simulink model "multi_opts"  (Simulink 4.00)
settings: Solver=ode45  SolverMode=SingleTasking  StartTime=0  StopTime=5  MaxStep=0.1  RelTol=1e-3  AbsTol=1e-3
libraries: simulink3 x3
(part 2 of 2)

== system multi_opts/GPe/2 input channel3/leaky integration ==
  Inport : Inport  Port=1  LatchInput=off
  Gain : Gain  Gain=A_rate  Multiplication=Element-wise(K.*u)  SaturateOnIntegerOverflow=on
  Integrator : Integrator  ExternalReset=none  InitialConditionSource=internal  InitialCondition=0  LimitOutput=off  UpperSaturationLimit=inf  LowerSaturationLimit=-inf  ShowSaturationPort=off  ShowStatePort=off  AbsoluteTolerance=auto
  decay const : Gain  Orientation=left  Gain=-A_rate  Multiplication=Element-wise(K.*u)  SaturateOnIntegerOverflow=on
  sum : Sum  Inputs=++  SaturateOnIntegerOverflow=on
  Outport : Outport  Port=1  InitialOutput=0
  wires:
  decay const/1 -> sum/2
  sum/1 -> Integrator/1
  Integrator/1 -> Outport/1, decay const/1
  Inport/1 -> Gain/1
  Gain/1 -> sum/1

== system multi_opts/GPe/2 input channel4/input summation ==
  x1 : Inport  Port=1  LatchInput=off
  x2 : Inport  Port=2  LatchInput=off
  Sum : Sum  Inputs=++  SaturateOnIntegerOverflow=on
  W1 : Gain  Gain=W_str  Multiplication=Element-wise(K.*u)  SaturateOnIntegerOverflow=on
  W2 : Gain  Gain=W_STN  Multiplication=Element-wise(K.*u)  SaturateOnIntegerOverflow=on
  out_1 : Outport  Port=1  InitialOutput=0
  wires:
  W2/1 -> Sum/2
  W1/1 -> Sum/1
  x2/1 -> W2/1
  x1/1 -> W1/1
  Sum/1 -> out_1/1

== system multi_opts/GPe/2 input channel4/leaky integration ==
  Inport : Inport  Port=1  LatchInput=off
  Gain : Gain  Gain=A_rate  Multiplication=Element-wise(K.*u)  SaturateOnIntegerOverflow=on
  Integrator : Integrator  ExternalReset=none  InitialConditionSource=internal  InitialCondition=0  LimitOutput=off  UpperSaturationLimit=inf  LowerSaturationLimit=-inf  ShowSaturationPort=off  ShowStatePort=off  AbsoluteTolerance=auto
  decay const : Gain  Orientation=left  Gain=-A_rate  Multiplication=Element-wise(K.*u)  SaturateOnIntegerOverflow=on
  sum : Sum  Inputs=++  SaturateOnIntegerOverflow=on
  Outport : Outport  Port=1  InitialOutput=0
  wires:
  Gain/1 -> sum/1
  Inport/1 -> Gain/1
  Integrator/1 -> decay const/1, Outport/1
  sum/1 -> Integrator/1
  decay const/1 -> sum/2

== system multi_opts/GPe/2 input channel5/input summation ==
  x1 : Inport  Port=1  LatchInput=off
  x2 : Inport  Port=2  LatchInput=off
  Sum : Sum  Inputs=++  SaturateOnIntegerOverflow=on
  W1 : Gain  Gain=W_str  Multiplication=Element-wise(K.*u)  SaturateOnIntegerOverflow=on
  W2 : Gain  Gain=W_STN  Multiplication=Element-wise(K.*u)  SaturateOnIntegerOverflow=on
  out_1 : Outport  Port=1  InitialOutput=0
  wires:
  Sum/1 -> out_1/1
  x1/1 -> W1/1
  x2/1 -> W2/1
  W1/1 -> Sum/1
  W2/1 -> Sum/2

== system multi_opts/GPe/2 input channel5/leaky integration ==
  Inport : Inport  Port=1  LatchInput=off
  Gain : Gain  Gain=A_rate  Multiplication=Element-wise(K.*u)  SaturateOnIntegerOverflow=on
  Integrator : Integrator  ExternalReset=none  InitialConditionSource=internal  InitialCondition=0  LimitOutput=off  UpperSaturationLimit=inf  LowerSaturationLimit=-inf  ShowSaturationPort=off  ShowStatePort=off  AbsoluteTolerance=auto
  decay const : Gain  Orientation=left  Gain=-A_rate  Multiplication=Element-wise(K.*u)  SaturateOnIntegerOverflow=on
  sum : Sum  Inputs=++  SaturateOnIntegerOverflow=on
  Outport : Outport  Port=1  InitialOutput=0
  wires:
  decay const/1 -> sum/2
  sum/1 -> Integrator/1
  Integrator/1 -> Outport/1, decay const/1
  Inport/1 -> Gain/1
  Gain/1 -> sum/1

== system multi_opts/GPi/2 input channel/input summation ==
  x1 : Inport  Port=1  LatchInput=off
  x2 : Inport  Port=2  LatchInput=off
  x3 : Inport  Port=3  LatchInput=off
  Sum : Sum  Inputs=+++  SaturateOnIntegerOverflow=on
  W1 : Gain  Gain=W_str  Multiplication=Element-wise(K.*u)  SaturateOnIntegerOverflow=on
  W2 : Gain  Gain=W_STN  Multiplication=Element-wise(K.*u)  SaturateOnIntegerOverflow=on
  W3 : Gain  Gain=W_GPe  Multiplication=Element-wise(K.*u)  SaturateOnIntegerOverflow=on
  out_1 : Outport  Port=1  InitialOutput=0
  wires:
  Sum/1 -> out_1/1
  x1/1 -> W1/1
  x2/1 -> W2/1
  W1/1 -> Sum/1
  W2/1 -> Sum/2
  x3/1 -> W3/1
  W3/1 -> Sum/3

== system multi_opts/GPi/2 input channel/leaky integration ==
  Inport : Inport  Port=1  LatchInput=off
  Gain : Gain  Gain=A_rate  Multiplication=Element-wise(K.*u)  SaturateOnIntegerOverflow=on
  Integrator : Integrator  ExternalReset=none  InitialConditionSource=internal  InitialCondition=0  LimitOutput=off  UpperSaturationLimit=inf  LowerSaturationLimit=-inf  ShowSaturationPort=off  ShowStatePort=off  AbsoluteTolerance=auto
  decay const : Gain  Orientation=left  Gain=-A_rate  Multiplication=Element-wise(K.*u)  SaturateOnIntegerOverflow=on
  sum : Sum  Inputs=++  SaturateOnIntegerOverflow=on
  Outport : Outport  Port=1  InitialOutput=0
  wires:
  decay const/1 -> sum/2
  sum/1 -> Integrator/1
  Integrator/1 -> Outport/1, decay const/1
  Inport/1 -> Gain/1
  Gain/1 -> sum/1

== system multi_opts/GPi/2 input channel1/input summation ==
  x1 : Inport  Port=1  LatchInput=off
  x2 : Inport  Port=2  LatchInput=off
  x3 : Inport  Port=3  LatchInput=off
  Sum : Sum  Inputs=+++  SaturateOnIntegerOverflow=on
  W1 : Gain  Gain=W_str  Multiplication=Element-wise(K.*u)  SaturateOnIntegerOverflow=on
  W2 : Gain  Gain=W_STN  Multiplication=Element-wise(K.*u)  SaturateOnIntegerOverflow=on
  W3 : Gain  Gain=W_GPe  Multiplication=Element-wise(K.*u)  SaturateOnIntegerOverflow=on
  out_1 : Outport  Port=1  InitialOutput=0
  wires:
  W3/1 -> Sum/3
  x3/1 -> W3/1
  W2/1 -> Sum/2
  W1/1 -> Sum/1
  x2/1 -> W2/1
  x1/1 -> W1/1
  Sum/1 -> out_1/1

== system multi_opts/GPi/2 input channel1/leaky integration ==
  Inport : Inport  Port=1  LatchInput=off
  Gain : Gain  Gain=A_rate  Multiplication=Element-wise(K.*u)  SaturateOnIntegerOverflow=on
  Integrator : Integrator  ExternalReset=none  InitialConditionSource=internal  InitialCondition=0  LimitOutput=off  UpperSaturationLimit=inf  LowerSaturationLimit=-inf  ShowSaturationPort=off  ShowStatePort=off  AbsoluteTolerance=auto
  decay const : Gain  Orientation=left  Gain=-A_rate  Multiplication=Element-wise(K.*u)  SaturateOnIntegerOverflow=on
  sum : Sum  Inputs=++  SaturateOnIntegerOverflow=on
  Outport : Outport  Port=1  InitialOutput=0
  wires:
  Gain/1 -> sum/1
  Inport/1 -> Gain/1
  Integrator/1 -> decay const/1, Outport/1
  sum/1 -> Integrator/1
  decay const/1 -> sum/2

== system multi_opts/GPi/2 input channel2/input summation ==
  x1 : Inport  Port=1  LatchInput=off
  x2 : Inport  Port=2  LatchInput=off
  x3 : Inport  Port=3  LatchInput=off
  Sum : Sum  Inputs=+++  SaturateOnIntegerOverflow=on
  W1 : Gain  Gain=W_str  Multiplication=Element-wise(K.*u)  SaturateOnIntegerOverflow=on
  W2 : Gain  Gain=W_STN  Multiplication=Element-wise(K.*u)  SaturateOnIntegerOverflow=on
  W3 : Gain  Gain=W_GPe  Multiplication=Element-wise(K.*u)  SaturateOnIntegerOverflow=on
  out_1 : Outport  Port=1  InitialOutput=0
  wires:
  Sum/1 -> out_1/1
  x1/1 -> W1/1
  x2/1 -> W2/1
  W1/1 -> Sum/1
  W2/1 -> Sum/2
  x3/1 -> W3/1
  W3/1 -> Sum/3

== system multi_opts/GPi/2 input channel2/leaky integration ==
  Inport : Inport  Port=1  LatchInput=off
  Gain : Gain  Gain=A_rate  Multiplication=Element-wise(K.*u)  SaturateOnIntegerOverflow=on
  Integrator : Integrator  ExternalReset=none  InitialConditionSource=internal  InitialCondition=0  LimitOutput=off  UpperSaturationLimit=inf  LowerSaturationLimit=-inf  ShowSaturationPort=off  ShowStatePort=off  AbsoluteTolerance=auto
  decay const : Gain  Orientation=left  Gain=-A_rate  Multiplication=Element-wise(K.*u)  SaturateOnIntegerOverflow=on
  sum : Sum  Inputs=++  SaturateOnIntegerOverflow=on
  Outport : Outport  Port=1  InitialOutput=0
  wires:
  decay const/1 -> sum/2
  sum/1 -> Integrator/1
  Integrator/1 -> Outport/1, decay const/1
  Inport/1 -> Gain/1
  Gain/1 -> sum/1

== system multi_opts/GPi/2 input channel3/input summation ==
  x1 : Inport  Port=1  LatchInput=off
  x2 : Inport  Port=2  LatchInput=off
  x3 : Inport  Port=3  LatchInput=off
  Sum : Sum  Inputs=+++  SaturateOnIntegerOverflow=on
  W1 : Gain  Gain=W_str  Multiplication=Element-wise(K.*u)  SaturateOnIntegerOverflow=on
  W2 : Gain  Gain=W_STN  Multiplication=Element-wise(K.*u)  SaturateOnIntegerOverflow=on
  W3 : Gain  Gain=W_GPe  Multiplication=Element-wise(K.*u)  SaturateOnIntegerOverflow=on
  out_1 : Outport  Port=1  InitialOutput=0
  wires:
  W3/1 -> Sum/3
  x3/1 -> W3/1
  W2/1 -> Sum/2
  W1/1 -> Sum/1
  x2/1 -> W2/1
  x1/1 -> W1/1
  Sum/1 -> out_1/1

== system multi_opts/GPi/2 input channel3/leaky integration ==
  Inport : Inport  Port=1  LatchInput=off
  Gain : Gain  Gain=A_rate  Multiplication=Element-wise(K.*u)  SaturateOnIntegerOverflow=on
  Integrator : Integrator  ExternalReset=none  InitialConditionSource=internal  InitialCondition=0  LimitOutput=off  UpperSaturationLimit=inf  LowerSaturationLimit=-inf  ShowSaturationPort=off  ShowStatePort=off  AbsoluteTolerance=auto
  decay const : Gain  Orientation=left  Gain=-A_rate  Multiplication=Element-wise(K.*u)  SaturateOnIntegerOverflow=on
  sum : Sum  Inputs=++  SaturateOnIntegerOverflow=on
  Outport : Outport  Port=1  InitialOutput=0
  wires:
  Gain/1 -> sum/1
  Inport/1 -> Gain/1
  Integrator/1 -> decay const/1, Outport/1
  sum/1 -> Integrator/1
  decay const/1 -> sum/2

== system multi_opts/GPi/2 input channel4/input summation ==
  x1 : Inport  Port=1  LatchInput=off
  x2 : Inport  Port=2  LatchInput=off
  x3 : Inport  Port=3  LatchInput=off
  Sum : Sum  Inputs=+++  SaturateOnIntegerOverflow=on
  W1 : Gain  Gain=W_str  Multiplication=Element-wise(K.*u)  SaturateOnIntegerOverflow=on
  W2 : Gain  Gain=W_STN  Multiplication=Element-wise(K.*u)  SaturateOnIntegerOverflow=on
  W3 : Gain  Gain=W_GPe  Multiplication=Element-wise(K.*u)  SaturateOnIntegerOverflow=on
  out_1 : Outport  Port=1  InitialOutput=0
  wires:
  Sum/1 -> out_1/1
  x1/1 -> W1/1
  x2/1 -> W2/1
  W1/1 -> Sum/1
  W2/1 -> Sum/2
  x3/1 -> W3/1
  W3/1 -> Sum/3

== system multi_opts/GPi/2 input channel4/leaky integration ==
  Inport : Inport  Port=1  LatchInput=off
  Gain : Gain  Gain=A_rate  Multiplication=Element-wise(K.*u)  SaturateOnIntegerOverflow=on
  Integrator : Integrator  ExternalReset=none  InitialConditionSource=internal  InitialCondition=0  LimitOutput=off  UpperSaturationLimit=inf  LowerSaturationLimit=-inf  ShowSaturationPort=off  ShowStatePort=off  AbsoluteTolerance=auto
  decay const : Gain  Orientation=left  Gain=-A_rate  Multiplication=Element-wise(K.*u)  SaturateOnIntegerOverflow=on
  sum : Sum  Inputs=++  SaturateOnIntegerOverflow=on
  Outport : Outport  Port=1  InitialOutput=0
  wires:
  decay const/1 -> sum/2
  sum/1 -> Integrator/1
  Integrator/1 -> Outport/1, decay const/1
  Inport/1 -> Gain/1
  Gain/1 -> sum/1

== system multi_opts/GPi/2 input channel5/input summation ==
  x1 : Inport  Port=1  LatchInput=off
  x2 : Inport  Port=2  LatchInput=off
  x3 : Inport  Port=3  LatchInput=off
  Sum : Sum  Inputs=+++  SaturateOnIntegerOverflow=on
  W1 : Gain  Gain=W_str  Multiplication=Element-wise(K.*u)  SaturateOnIntegerOverflow=on
  W2 : Gain  Gain=W_STN  Multiplication=Element-wise(K.*u)  SaturateOnIntegerOverflow=on
  W3 : Gain  Gain=W_GPe  Multiplication=Element-wise(K.*u)  SaturateOnIntegerOverflow=on
  out_1 : Outport  Port=1  InitialOutput=0
  wires:
  W3/1 -> Sum/3
  x3/1 -> W3/1
  W2/1 -> Sum/2
  W1/1 -> Sum/1
  x2/1 -> W2/1
  x1/1 -> W1/1
  Sum/1 -> out_1/1

== system multi_opts/GPi/2 input channel5/leaky integration ==
  Inport : Inport  Port=1  LatchInput=off
  Gain : Gain  Gain=A_rate  Multiplication=Element-wise(K.*u)  SaturateOnIntegerOverflow=on
  Integrator : Integrator  ExternalReset=none  InitialConditionSource=internal  InitialCondition=0  LimitOutput=off  UpperSaturationLimit=inf  LowerSaturationLimit=-inf  ShowSaturationPort=off  ShowStatePort=off  AbsoluteTolerance=auto
  decay const : Gain  Orientation=left  Gain=-A_rate  Multiplication=Element-wise(K.*u)  SaturateOnIntegerOverflow=on
  sum : Sum  Inputs=++  SaturateOnIntegerOverflow=on
  Outport : Outport  Port=1  InitialOutput=0
  wires:
  Gain/1 -> sum/1
  Inport/1 -> Gain/1
  Integrator/1 -> decay const/1, Outport/1
  sum/1 -> Integrator/1
  decay const/1 -> sum/2

== system multi_opts/STN/STN discrete model/2 input channel ==
  Cortex : Inport  Orientation=down  Port=1  LatchInput=off
  GPe : Inport  Orientation=down  Port=2  LatchInput=off
  input summation : Subsystem  Orientation=down
      settings: RTWFcnNameOpts=Auto  RTWFileNameOpts=Auto
  leaky integration : Subsystem  Orientation=down
      settings: RTWFcnNameOpts=Auto  RTWFileNameOpts=Auto
  piecewise lin. : S-Function  Orientation=down  FunctionName=Mpieclin  Parameters=slope,thresh  PortCounts=[]  SFunctionModules=''
  out : Outport  Orientation=down  Port=1  InitialOutput=0
  wires:
  piecewise lin./1 -> out/1
  GPe/1 -> input summation/2(x2)
  Cortex/1 -> input summation/1(x1)
  leaky integration/1(Outport) -> piecewise lin./1
  input summation/1(out_1) -> leaky integration/1(Inport)

== system multi_opts/STN/STN discrete model/2 input channel1 ==
  Cortex : Inport  Orientation=down  Port=1  LatchInput=off
  GPe : Inport  Orientation=down  Port=2  LatchInput=off
  input summation : Subsystem  Orientation=down
      settings: RTWFcnNameOpts=Auto  RTWFileNameOpts=Auto
  leaky integration : Subsystem  Orientation=down
      settings: RTWFcnNameOpts=Auto  RTWFileNameOpts=Auto
  piecewise lin. : S-Function  Orientation=down  FunctionName=Mpieclin  Parameters=slope,thresh  PortCounts=[]  SFunctionModules=''
  out : Outport  Orientation=down  Port=1  InitialOutput=0
  wires:
  input summation/1(out_1) -> leaky integration/1(Inport)
  leaky integration/1(Outport) -> piecewise lin./1
  Cortex/1 -> input summation/1(x1)
  GPe/1 -> input summation/2(x2)
  piecewise lin./1 -> out/1

== system multi_opts/STN/STN discrete model/2 input channel2 ==
  Cortex : Inport  Orientation=down  Port=1  LatchInput=off
  GPe : Inport  Orientation=down  Port=2  LatchInput=off
  input summation : Subsystem  Orientation=down
      settings: RTWFcnNameOpts=Auto  RTWFileNameOpts=Auto
  leaky integration : Subsystem  Orientation=down
      settings: RTWFcnNameOpts=Auto  RTWFileNameOpts=Auto
  piecewise lin. : S-Function  Orientation=down  FunctionName=Mpieclin  Parameters=slope,thresh  PortCounts=[]  SFunctionModules=''
  out : Outport  Orientation=down  Port=1  InitialOutput=0
  wires:
  piecewise lin./1 -> out/1
  GPe/1 -> input summation/2(x2)
  Cortex/1 -> input summation/1(x1)
  leaky integration/1(Outport) -> piecewise lin./1
  input summation/1(out_1) -> leaky integration/1(Inport)

== system multi_opts/STN/STN discrete model/2 input channel3 ==
  Cortex : Inport  Orientation=down  Port=1  LatchInput=off
  GPe : Inport  Orientation=down  Port=2  LatchInput=off
  input summation : Subsystem  Orientation=down
      settings: RTWFcnNameOpts=Auto  RTWFileNameOpts=Auto
  leaky integration : Subsystem  Orientation=down
      settings: RTWFcnNameOpts=Auto  RTWFileNameOpts=Auto
  piecewise lin. : S-Function  Orientation=down  FunctionName=Mpieclin  Parameters=slope,thresh  PortCounts=[]  SFunctionModules=''
  out : Outport  Orientation=down  Port=1  InitialOutput=0
  wires:
  input summation/1(out_1) -> leaky integration/1(Inport)
  leaky integration/1(Outport) -> piecewise lin./1
  Cortex/1 -> input summation/1(x1)
  GPe/1 -> input summation/2(x2)
  piecewise lin./1 -> out/1

== system multi_opts/STN/STN discrete model/2 input channel4 ==
  Cortex : Inport  Orientation=down  Port=1  LatchInput=off
  GPe : Inport  Orientation=down  Port=2  LatchInput=off
  input summation : Subsystem  Orientation=down
      settings: RTWFcnNameOpts=Auto  RTWFileNameOpts=Auto
  leaky integration : Subsystem  Orientation=down
      settings: RTWFcnNameOpts=Auto  RTWFileNameOpts=Auto
  piecewise lin. : S-Function  Orientation=down  FunctionName=Mpieclin  Parameters=slope,thresh  PortCounts=[]  SFunctionModules=''
  out : Outport  Orientation=down  Port=1  InitialOutput=0
  wires:
  piecewise lin./1 -> out/1
  GPe/1 -> input summation/2(x2)
  Cortex/1 -> input summation/1(x1)
  leaky integration/1(Outport) -> piecewise lin./1
  input summation/1(out_1) -> leaky integration/1(Inport)

== system multi_opts/STN/STN discrete model/2 input channel5 ==
  Cortex : Inport  Orientation=down  Port=1  LatchInput=off
  GPe : Inport  Orientation=down  Port=2  LatchInput=off
  input summation : Subsystem  Orientation=down
      settings: RTWFcnNameOpts=Auto  RTWFileNameOpts=Auto
  leaky integration : Subsystem  Orientation=down
      settings: RTWFcnNameOpts=Auto  RTWFileNameOpts=Auto
  piecewise lin. : S-Function  Orientation=down  FunctionName=Mpieclin  Parameters=slope,thresh  PortCounts=[]  SFunctionModules=''
  out : Outport  Orientation=down  Port=1  InitialOutput=0
  wires:
  input summation/1(out_1) -> leaky integration/1(Inport)
  leaky integration/1(Outport) -> piecewise lin./1
  Cortex/1 -> input summation/1(x1)
  GPe/1 -> input summation/2(x2)
  piecewise lin./1 -> out/1

== system multi_opts/STN/STN homogeneous model/3 input channel ==
  Cortex : Inport  Orientation=down  Port=1  LatchInput=off
  GPe : Inport  Orientation=down  Port=2  LatchInput=off
  Tonic Ctx : Inport  Orientation=down  Port=3  LatchInput=off
  input summation : Subsystem  Orientation=down
      settings: RTWFcnNameOpts=Auto  RTWFileNameOpts=Auto
  leaky integration : Subsystem  Orientation=down
      settings: RTWFcnNameOpts=Auto  RTWFileNameOpts=Auto
  piecewise lin. : S-Function  Orientation=down  FunctionName=Mpieclin  Parameters=slope,thresh  PortCounts=[]  SFunctionModules=''
  out : Outport  Orientation=down  Port=1  InitialOutput=0
  wires:
  leaky integration/1(Outport) -> piecewise lin./1
  Cortex/1 -> input summation/1(x1)
  GPe/1 -> input summation/2(x2)
  Tonic Ctx/1 -> input summation/3(x3)
  input summation/1(out_1) -> leaky integration/1(Inport)
  piecewise lin./1 -> out/1

== system multi_opts/Striatum(D1)/chan1/leaky integration ==
  Inport : Inport  Port=1  LatchInput=off  PortDimensions=1
  Gain : Gain  Gain=A_rate  Multiplication=Element-wise(K.*u)  SaturateOnIntegerOverflow=on
  Integrator : Integrator  ExternalReset=none  InitialConditionSource=internal  InitialCondition=0  LimitOutput=off  UpperSaturationLimit=inf  LowerSaturationLimit=-inf  ShowSaturationPort=off  ShowStatePort=off  AbsoluteTolerance=auto
  decay const : Gain  Orientation=left  Gain=-A_rate  Multiplication=Element-wise(K.*u)  SaturateOnIntegerOverflow=on
  sum : Sum  Inputs=++  SaturateOnIntegerOverflow=on
  Outport : Outport  Port=1  InitialOutput=0
  wires:
  decay const/1 -> sum/2
  sum/1 -> Integrator/1
  Integrator/1 -> decay const/1, Outport/1
  Inport/1 -> Gain/1
  Gain/1 -> sum/1

== system multi_opts/Striatum(D1)/chan2/leaky integration ==
  Inport : Inport  Port=1  LatchInput=off
  Gain : Gain  Gain=A_rate  Multiplication=Element-wise(K.*u)  SaturateOnIntegerOverflow=on
  Integrator : Integrator  ExternalReset=none  InitialConditionSource=internal  InitialCondition=0  LimitOutput=off  UpperSaturationLimit=inf  LowerSaturationLimit=-inf  ShowSaturationPort=off  ShowStatePort=off  AbsoluteTolerance=auto
  decay const : Gain  Orientation=left  Gain=-A_rate  Multiplication=Element-wise(K.*u)  SaturateOnIntegerOverflow=on
  sum : Sum  Inputs=++  SaturateOnIntegerOverflow=on
  Outport : Outport  Port=1  InitialOutput=0
  wires:
  Gain/1 -> sum/1
  Inport/1 -> Gain/1
  Integrator/1 -> Outport/1, decay const/1
  sum/1 -> Integrator/1
  decay const/1 -> sum/2

== system multi_opts/Striatum(D1)/chan3/leaky integration ==
  Inport : Inport  Port=1  LatchInput=off
  Gain : Gain  Gain=A_rate  Multiplication=Element-wise(K.*u)  SaturateOnIntegerOverflow=on
  Integrator : Integrator  ExternalReset=none  InitialConditionSource=internal  InitialCondition=0  LimitOutput=off  UpperSaturationLimit=inf  LowerSaturationLimit=-inf  ShowSaturationPort=off  ShowStatePort=off  AbsoluteTolerance=auto
  decay const : Gain  Orientation=left  Gain=-A_rate  Multiplication=Element-wise(K.*u)  SaturateOnIntegerOverflow=on
  sum : Sum  Inputs=++  SaturateOnIntegerOverflow=on
  Outport : Outport  Port=1  InitialOutput=0
  wires:
  decay const/1 -> sum/2
  sum/1 -> Integrator/1
  Integrator/1 -> decay const/1, Outport/1
  Inport/1 -> Gain/1
  Gain/1 -> sum/1

== system multi_opts/Striatum(D1)/chan4/leaky integration ==
  Inport : Inport  Port=1  LatchInput=off  PortDimensions=1
  Gain : Gain  Gain=A_rate  Multiplication=Element-wise(K.*u)  SaturateOnIntegerOverflow=on
  Integrator : Integrator  ExternalReset=none  InitialConditionSource=internal  InitialCondition=0  LimitOutput=off  UpperSaturationLimit=inf  LowerSaturationLimit=-inf  ShowSaturationPort=off  ShowStatePort=off  AbsoluteTolerance=auto
  decay const : Gain  Orientation=left  Gain=-A_rate  Multiplication=Element-wise(K.*u)  SaturateOnIntegerOverflow=on
  sum : Sum  Inputs=++  SaturateOnIntegerOverflow=on
  Outport : Outport  Port=1  InitialOutput=0
  wires:
  Gain/1 -> sum/1
  Inport/1 -> Gain/1
  Integrator/1 -> Outport/1, decay const/1
  sum/1 -> Integrator/1
  decay const/1 -> sum/2

== system multi_opts/Striatum(D1)/chan5/leaky integration ==
  Inport : Inport  Port=1  LatchInput=off
  Gain : Gain  Gain=A_rate  Multiplication=Element-wise(K.*u)  SaturateOnIntegerOverflow=on
  Integrator : Integrator  ExternalReset=none  InitialConditionSource=internal  InitialCondition=0  LimitOutput=off  UpperSaturationLimit=inf  LowerSaturationLimit=-inf  ShowSaturationPort=off  ShowStatePort=off  AbsoluteTolerance=auto
  decay const : Gain  Orientation=left  Gain=-A_rate  Multiplication=Element-wise(K.*u)  SaturateOnIntegerOverflow=on
  sum : Sum  Inputs=++  SaturateOnIntegerOverflow=on
  Outport : Outport  Port=1  InitialOutput=0
  wires:
  decay const/1 -> sum/2
  sum/1 -> Integrator/1
  Integrator/1 -> decay const/1, Outport/1
  Inport/1 -> Gain/1
  Gain/1 -> sum/1

== system multi_opts/Striatum(D1)/chan6/leaky integration ==
  Inport : Inport  Port=1  LatchInput=off
  Gain : Gain  Gain=A_rate  Multiplication=Element-wise(K.*u)  SaturateOnIntegerOverflow=on
  Integrator : Integrator  ExternalReset=none  InitialConditionSource=internal  InitialCondition=0  LimitOutput=off  UpperSaturationLimit=inf  LowerSaturationLimit=-inf  ShowSaturationPort=off  ShowStatePort=off  AbsoluteTolerance=auto
  decay const : Gain  Orientation=left  Gain=-A_rate  Multiplication=Element-wise(K.*u)  SaturateOnIntegerOverflow=on
  sum : Sum  Inputs=++  SaturateOnIntegerOverflow=on
  Outport : Outport  Port=1  InitialOutput=0
  wires:
  Gain/1 -> sum/1
  Inport/1 -> Gain/1
  Integrator/1 -> Outport/1, decay const/1
  sum/1 -> Integrator/1
  decay const/1 -> sum/2

== system multi_opts/Striatum(D2)/chan1/leaky integration ==
  Inport : Inport  Port=1  LatchInput=off  PortDimensions=1
  Gain : Gain  Gain=A_rate  Multiplication=Element-wise(K.*u)  SaturateOnIntegerOverflow=on
  Integrator : Integrator  ExternalReset=none  InitialConditionSource=internal  InitialCondition=0  LimitOutput=off  UpperSaturationLimit=inf  LowerSaturationLimit=-inf  ShowSaturationPort=off  ShowStatePort=off  AbsoluteTolerance=auto
  decay const : Gain  Orientation=left  Gain=-A_rate  Multiplication=Element-wise(K.*u)  SaturateOnIntegerOverflow=on
  sum : Sum  Inputs=++  SaturateOnIntegerOverflow=on
  Outport : Outport  Port=1  InitialOutput=0
  wires:
  Gain/1 -> sum/1
  Inport/1 -> Gain/1
  Integrator/1 -> Outport/1, decay const/1
  sum/1 -> Integrator/1
  decay const/1 -> sum/2

== system multi_opts/Striatum(D2)/chan2/leaky integration ==
  Inport : Inport  Port=1  LatchInput=off  PortDimensions=1
  Gain : Gain  Gain=A_rate  Multiplication=Element-wise(K.*u)  SaturateOnIntegerOverflow=on
  Integrator : Integrator  ExternalReset=none  InitialConditionSource=internal  InitialCondition=0  LimitOutput=off  UpperSaturationLimit=inf  LowerSaturationLimit=-inf  ShowSaturationPort=off  ShowStatePort=off  AbsoluteTolerance=auto
  decay const : Gain  Orientation=left  Gain=-A_rate  Multiplication=Element-wise(K.*u)  SaturateOnIntegerOverflow=on
  sum : Sum  Inputs=++  SaturateOnIntegerOverflow=on
  Outport : Outport  Port=1  InitialOutput=0
  wires:
  decay const/1 -> sum/2
  sum/1 -> Integrator/1
  Integrator/1 -> decay const/1, Outport/1
  Inport/1 -> Gain/1
  Gain/1 -> sum/1

== system multi_opts/Striatum(D2)/chan3/leaky integration ==
  Inport : Inport  Port=1  LatchInput=off  PortDimensions=1
  Gain : Gain  Gain=A_rate  Multiplication=Element-wise(K.*u)  SaturateOnIntegerOverflow=on
  Integrator : Integrator  ExternalReset=none  InitialConditionSource=internal  InitialCondition=0  LimitOutput=off  UpperSaturationLimit=inf  LowerSaturationLimit=-inf  ShowSaturationPort=off  ShowStatePort=off  AbsoluteTolerance=auto
  decay const : Gain  Orientation=left  Gain=-A_rate  Multiplication=Element-wise(K.*u)  SaturateOnIntegerOverflow=on
  sum : Sum  Inputs=++  SaturateOnIntegerOverflow=on
  Outport : Outport  Port=1  InitialOutput=0
  wires:
  Gain/1 -> sum/1
  Inport/1 -> Gain/1
  Integrator/1 -> Outport/1, decay const/1
  sum/1 -> Integrator/1
  decay const/1 -> sum/2

== system multi_opts/Striatum(D2)/chan4/leaky integration ==
  Inport : Inport  Port=1  LatchInput=off  PortDimensions=1
  Gain : Gain  Gain=A_rate  Multiplication=Element-wise(K.*u)  SaturateOnIntegerOverflow=on
  Integrator : Integrator  ExternalReset=none  InitialConditionSource=internal  InitialCondition=0  LimitOutput=off  UpperSaturationLimit=inf  LowerSaturationLimit=-inf  ShowSaturationPort=off  ShowStatePort=off  AbsoluteTolerance=auto
  decay const : Gain  Orientation=left  Gain=-A_rate  Multiplication=Element-wise(K.*u)  SaturateOnIntegerOverflow=on
  sum : Sum  Inputs=++  SaturateOnIntegerOverflow=on
  Outport : Outport  Port=1  InitialOutput=0
  wires:
  decay const/1 -> sum/2
  sum/1 -> Integrator/1
  Integrator/1 -> decay const/1, Outport/1
  Inport/1 -> Gain/1
  Gain/1 -> sum/1

== system multi_opts/Striatum(D2)/chan5/leaky integration ==
  Inport : Inport  Port=1  LatchInput=off  PortDimensions=1
  Gain : Gain  Gain=A_rate  Multiplication=Element-wise(K.*u)  SaturateOnIntegerOverflow=on
  Integrator : Integrator  ExternalReset=none  InitialConditionSource=internal  InitialCondition=0  LimitOutput=off  UpperSaturationLimit=inf  LowerSaturationLimit=-inf  ShowSaturationPort=off  ShowStatePort=off  AbsoluteTolerance=auto
  decay const : Gain  Orientation=left  Gain=-A_rate  Multiplication=Element-wise(K.*u)  SaturateOnIntegerOverflow=on
  sum : Sum  Inputs=++  SaturateOnIntegerOverflow=on
  Outport : Outport  Port=1  InitialOutput=0
  wires:
  Gain/1 -> sum/1
  Inport/1 -> Gain/1
  Integrator/1 -> Outport/1, decay const/1
  sum/1 -> Integrator/1
  decay const/1 -> sum/2

== system multi_opts/Striatum(D2)/chan6/leaky integration ==
  Inport : Inport  Port=1  LatchInput=off  PortDimensions=1
  Gain : Gain  Gain=A_rate  Multiplication=Element-wise(K.*u)  SaturateOnIntegerOverflow=on
  Integrator : Integrator  ExternalReset=none  InitialConditionSource=internal  InitialCondition=0  LimitOutput=off  UpperSaturationLimit=inf  LowerSaturationLimit=-inf  ShowSaturationPort=off  ShowStatePort=off  AbsoluteTolerance=auto
  decay const : Gain  Orientation=left  Gain=-A_rate  Multiplication=Element-wise(K.*u)  SaturateOnIntegerOverflow=on
  sum : Sum  Inputs=++  SaturateOnIntegerOverflow=on
  Outport : Outport  Port=1  InitialOutput=0
  wires:
  decay const/1 -> sum/2
  sum/1 -> Integrator/1
  Integrator/1 -> decay const/1, Outport/1
  Inport/1 -> Gain/1
  Gain/1 -> sum/1

== system multi_opts/STN/STN discrete model/2 input channel/input summation ==
  x1 : Inport  Port=1  LatchInput=off
  x2 : Inport  Port=2  LatchInput=off
  Sum : Sum  Inputs=++  SaturateOnIntegerOverflow=on
  W1 : Gain  Gain=W_ctx  Multiplication=Element-wise(K.*u)  SaturateOnIntegerOverflow=on
  W2 : Gain  Gain=W_GPe  Multiplication=Element-wise(K.*u)  SaturateOnIntegerOverflow=on
  out_1 : Outport  Port=1  InitialOutput=0
  wires:
  Sum/1 -> out_1/1
  x1/1 -> W1/1
  x2/1 -> W2/1
  W1/1 -> Sum/1
  W2/1 -> Sum/2

== system multi_opts/STN/STN discrete model/2 input channel/leaky integration ==
  Inport : Inport  Port=1  LatchInput=off
  Gain : Gain  Gain=A_rate  Multiplication=Element-wise(K.*u)  SaturateOnIntegerOverflow=on
  Integrator : Integrator  ExternalReset=none  InitialConditionSource=internal  InitialCondition=0  LimitOutput=off  UpperSaturationLimit=inf  LowerSaturationLimit=-inf  ShowSaturationPort=off  ShowStatePort=off  AbsoluteTolerance=auto
  decay const : Gain  Orientation=left  Gain=-A_rate  Multiplication=Element-wise(K.*u)  SaturateOnIntegerOverflow=on
  sum : Sum  Inputs=++  SaturateOnIntegerOverflow=on
  Outport : Outport  Port=1  InitialOutput=0
  wires:
  decay const/1 -> sum/2
  sum/1 -> Integrator/1
  Integrator/1 -> Outport/1, decay const/1
  Inport/1 -> Gain/1
  Gain/1 -> sum/1

== system multi_opts/STN/STN discrete model/2 input channel1/input summation ==
  x1 : Inport  Port=1  LatchInput=off
  x2 : Inport  Port=2  LatchInput=off
  Sum : Sum  Inputs=++  SaturateOnIntegerOverflow=on
  W1 : Gain  Gain=W_ctx  Multiplication=Element-wise(K.*u)  SaturateOnIntegerOverflow=on
  W2 : Gain  Gain=W_GPe  Multiplication=Element-wise(K.*u)  SaturateOnIntegerOverflow=on
  out_1 : Outport  Port=1  InitialOutput=0
  wires:
  W2/1 -> Sum/2
  W1/1 -> Sum/1
  x2/1 -> W2/1
  x1/1 -> W1/1
  Sum/1 -> out_1/1

== system multi_opts/STN/STN discrete model/2 input channel1/leaky integration ==
  Inport : Inport  Port=1  LatchInput=off
  Gain : Gain  Gain=A_rate  Multiplication=Element-wise(K.*u)  SaturateOnIntegerOverflow=on
  Integrator : Integrator  ExternalReset=none  InitialConditionSource=internal  InitialCondition=0  LimitOutput=off  UpperSaturationLimit=inf  LowerSaturationLimit=-inf  ShowSaturationPort=off  ShowStatePort=off  AbsoluteTolerance=auto
  decay const : Gain  Orientation=left  Gain=-A_rate  Multiplication=Element-wise(K.*u)  SaturateOnIntegerOverflow=on
  sum : Sum  Inputs=++  SaturateOnIntegerOverflow=on
  Outport : Outport  Port=1  InitialOutput=0
  wires:
  Gain/1 -> sum/1
  Inport/1 -> Gain/1
  Integrator/1 -> decay const/1, Outport/1
  sum/1 -> Integrator/1
  decay const/1 -> sum/2

== system multi_opts/STN/STN discrete model/2 input channel2/input summation ==
  x1 : Inport  Port=1  LatchInput=off
  x2 : Inport  Port=2  LatchInput=off
  Sum : Sum  Inputs=++  SaturateOnIntegerOverflow=on
  W1 : Gain  Gain=W_ctx  Multiplication=Element-wise(K.*u)  SaturateOnIntegerOverflow=on
  W2 : Gain  Gain=W_GPe  Multiplication=Element-wise(K.*u)  SaturateOnIntegerOverflow=on
  out_1 : Outport  Port=1  InitialOutput=0
  wires:
  Sum/1 -> out_1/1
  x1/1 -> W1/1
  x2/1 -> W2/1
  W1/1 -> Sum/1
  W2/1 -> Sum/2

== system multi_opts/STN/STN discrete model/2 input channel2/leaky integration ==
  Inport : Inport  Port=1  LatchInput=off
  Gain : Gain  Gain=A_rate  Multiplication=Element-wise(K.*u)  SaturateOnIntegerOverflow=on
  Integrator : Integrator  ExternalReset=none  InitialConditionSource=internal  InitialCondition=0  LimitOutput=off  UpperSaturationLimit=inf  LowerSaturationLimit=-inf  ShowSaturationPort=off  ShowStatePort=off  AbsoluteTolerance=auto
  decay const : Gain  Orientation=left  Gain=-A_rate  Multiplication=Element-wise(K.*u)  SaturateOnIntegerOverflow=on
  sum : Sum  Inputs=++  SaturateOnIntegerOverflow=on
  Outport : Outport  Port=1  InitialOutput=0
  wires:
  decay const/1 -> sum/2
  sum/1 -> Integrator/1
  Integrator/1 -> Outport/1, decay const/1
  Inport/1 -> Gain/1
  Gain/1 -> sum/1

== system multi_opts/STN/STN discrete model/2 input channel3/input summation ==
  x1 : Inport  Port=1  LatchInput=off
  x2 : Inport  Port=2  LatchInput=off
  Sum : Sum  Inputs=++  SaturateOnIntegerOverflow=on
  W1 : Gain  Gain=W_ctx  Multiplication=Element-wise(K.*u)  SaturateOnIntegerOverflow=on
  W2 : Gain  Gain=W_GPe  Multiplication=Element-wise(K.*u)  SaturateOnIntegerOverflow=on
  out_1 : Outport  Port=1  InitialOutput=0
  wires:
  W2/1 -> Sum/2
  W1/1 -> Sum/1
  x2/1 -> W2/1
  x1/1 -> W1/1
  Sum/1 -> out_1/1

== system multi_opts/STN/STN discrete model/2 input channel3/leaky integration ==
  Inport : Inport  Port=1  LatchInput=off
  Gain : Gain  Gain=A_rate  Multiplication=Element-wise(K.*u)  SaturateOnIntegerOverflow=on
  Integrator : Integrator  ExternalReset=none  InitialConditionSource=internal  InitialCondition=0  LimitOutput=off  UpperSaturationLimit=inf  LowerSaturationLimit=-inf  ShowSaturationPort=off  ShowStatePort=off  AbsoluteTolerance=auto
  decay const : Gain  Orientation=left  Gain=-A_rate  Multiplication=Element-wise(K.*u)  SaturateOnIntegerOverflow=on
  sum : Sum  Inputs=++  SaturateOnIntegerOverflow=on
  Outport : Outport  Port=1  InitialOutput=0
  wires:
  Gain/1 -> sum/1
  Inport/1 -> Gain/1
  Integrator/1 -> decay const/1, Outport/1
  sum/1 -> Integrator/1
  decay const/1 -> sum/2

== system multi_opts/STN/STN discrete model/2 input channel4/input summation ==
  x1 : Inport  Port=1  LatchInput=off
  x2 : Inport  Port=2  LatchInput=off
  Sum : Sum  Inputs=++  SaturateOnIntegerOverflow=on
  W1 : Gain  Gain=W_ctx  Multiplication=Element-wise(K.*u)  SaturateOnIntegerOverflow=on
  W2 : Gain  Gain=W_GPe  Multiplication=Element-wise(K.*u)  SaturateOnIntegerOverflow=on
  out_1 : Outport  Port=1  InitialOutput=0
  wires:
  Sum/1 -> out_1/1
  x1/1 -> W1/1
  x2/1 -> W2/1
  W1/1 -> Sum/1
  W2/1 -> Sum/2

== system multi_opts/STN/STN discrete model/2 input channel4/leaky integration ==
  Inport : Inport  Port=1  LatchInput=off
  Gain : Gain  Gain=A_rate  Multiplication=Element-wise(K.*u)  SaturateOnIntegerOverflow=on
  Integrator : Integrator  ExternalReset=none  InitialConditionSource=internal  InitialCondition=0  LimitOutput=off  UpperSaturationLimit=inf  LowerSaturationLimit=-inf  ShowSaturationPort=off  ShowStatePort=off  AbsoluteTolerance=auto
  decay const : Gain  Orientation=left  Gain=-A_rate  Multiplication=Element-wise(K.*u)  SaturateOnIntegerOverflow=on
  sum : Sum  Inputs=++  SaturateOnIntegerOverflow=on
  Outport : Outport  Port=1  InitialOutput=0
  wires:
  decay const/1 -> sum/2
  sum/1 -> Integrator/1
  Integrator/1 -> Outport/1, decay const/1
  Inport/1 -> Gain/1
  Gain/1 -> sum/1

== system multi_opts/STN/STN discrete model/2 input channel5/input summation ==
  x1 : Inport  Port=1  LatchInput=off
  x2 : Inport  Port=2  LatchInput=off
  Sum : Sum  Inputs=++  SaturateOnIntegerOverflow=on
  W1 : Gain  Gain=W_ctx  Multiplication=Element-wise(K.*u)  SaturateOnIntegerOverflow=on
  W2 : Gain  Gain=W_GPe  Multiplication=Element-wise(K.*u)  SaturateOnIntegerOverflow=on
  out_1 : Outport  Port=1  InitialOutput=0
  wires:
  W2/1 -> Sum/2
  W1/1 -> Sum/1
  x2/1 -> W2/1
  x1/1 -> W1/1
  Sum/1 -> out_1/1

== system multi_opts/STN/STN discrete model/2 input channel5/leaky integration ==
  Inport : Inport  Port=1  LatchInput=off
  Gain : Gain  Gain=A_rate  Multiplication=Element-wise(K.*u)  SaturateOnIntegerOverflow=on
  Integrator : Integrator  ExternalReset=none  InitialConditionSource=internal  InitialCondition=0  LimitOutput=off  UpperSaturationLimit=inf  LowerSaturationLimit=-inf  ShowSaturationPort=off  ShowStatePort=off  AbsoluteTolerance=auto
  decay const : Gain  Orientation=left  Gain=-A_rate  Multiplication=Element-wise(K.*u)  SaturateOnIntegerOverflow=on
  sum : Sum  Inputs=++  SaturateOnIntegerOverflow=on
  Outport : Outport  Port=1  InitialOutput=0
  wires:
  Gain/1 -> sum/1
  Inport/1 -> Gain/1
  Integrator/1 -> decay const/1, Outport/1
  sum/1 -> Integrator/1
  decay const/1 -> sum/2

== system multi_opts/STN/STN homogeneous model/3 input channel/input summation ==
  x1 : Inport  Port=1  LatchInput=off
  x2 : Inport  Port=2  LatchInput=off
  x3 : Inport  Port=3  LatchInput=off
  Sum : Sum  Inputs=+++  SaturateOnIntegerOverflow=on
  W1 : Gain  Gain=W_ctx  Multiplication=Element-wise(K.*u)  SaturateOnIntegerOverflow=on
  W2 : Gain  Gain=W_GPe  Multiplication=Element-wise(K.*u)  SaturateOnIntegerOverflow=on
  W3 : Gain  Gain=1  Multiplication=Element-wise(K.*u)  SaturateOnIntegerOverflow=on
  out_1 : Outport  Port=1  InitialOutput=0
  wires:
  W3/1 -> Sum/3
  x3/1 -> W3/1
  W2/1 -> Sum/2
  W1/1 -> Sum/1
  x2/1 -> W2/1
  x1/1 -> W1/1
  Sum/1 -> out_1/1

== system multi_opts/STN/STN homogeneous model/3 input channel/leaky integration ==
  Inport : Inport  Port=1  LatchInput=off
  Gain : Gain  Gain=A_rate  Multiplication=Element-wise(K.*u)  SaturateOnIntegerOverflow=on
  Integrator : Integrator  ExternalReset=none  InitialConditionSource=internal  InitialCondition=0  LimitOutput=off  UpperSaturationLimit=inf  LowerSaturationLimit=-inf  ShowSaturationPort=off  ShowStatePort=off  AbsoluteTolerance=auto
  decay const : Gain  Orientation=left  Gain=-A_rate  Multiplication=Element-wise(K.*u)  SaturateOnIntegerOverflow=on
  sum : Sum  Inputs=++  SaturateOnIntegerOverflow=on
  Outport : Outport  Port=1  InitialOutput=0
  wires:
  Gain/1 -> sum/1
  Inport/1 -> Gain/1
  Integrator/1 -> decay const/1, Outport/1
  sum/1 -> Integrator/1
  decay const/1 -> sum/2
